simulink model "AWD_EV_MODEL_rev2"  (Simulink 8.7)
settings: Solver=ode3  SolverMode=SingleTasking  StartTime=0.0  StopTime=20  FixedStep=0.001  RelTol=1e-3
undefined symbols (not defined in the file): Bx, Bx_2, By, By_2, Cx, Cx_2, Cy, Cy_2, Dx, Dx_2, Dy, Dy_2, Ex, Ex_2, Ey, Ey_2, g, GRR, GRR_E, hg, Ixx, Iyy, Jw, Jz, Lf, Lr, Lw, m, r0, Rw, rx1, rx1_2, rx2, rx2_2, ry1, ry1_2, ry2, ry2_2, SA_A, SA_SAT_n, SA_SAT_p, SA_Slope, sigbuilder_block, Split_u_Time_On, SR_Eq_Accel_Brake_Threshold, Steering_Input_Select, T_Avail, Throttle_Final_Val, Throttle_Init_Val, Throttle_Step_Time, Vx0, Vy0, wRL0, z
libraries: simulink x10
(part 1 of 2)
settings Model: Creator=ETLAB  LastModifiedBy=MR Spyder
settings DataIOCC: SignalLoggingSaveFormat=ModelDataLogs
settings OptimizationCC: ExpressionDepthLimit=2147483647
settings DebuggingCC: SolverPrmCheckMsg=warning  InheritedTsInSrcMsg=none  FcnCallInpInsideContextMsg=EnableAllAsWarning  StateNameClashWarn=warning
settings GRTTargetCC: CombineOutputUpdateFcns=off  GRTInterface=on

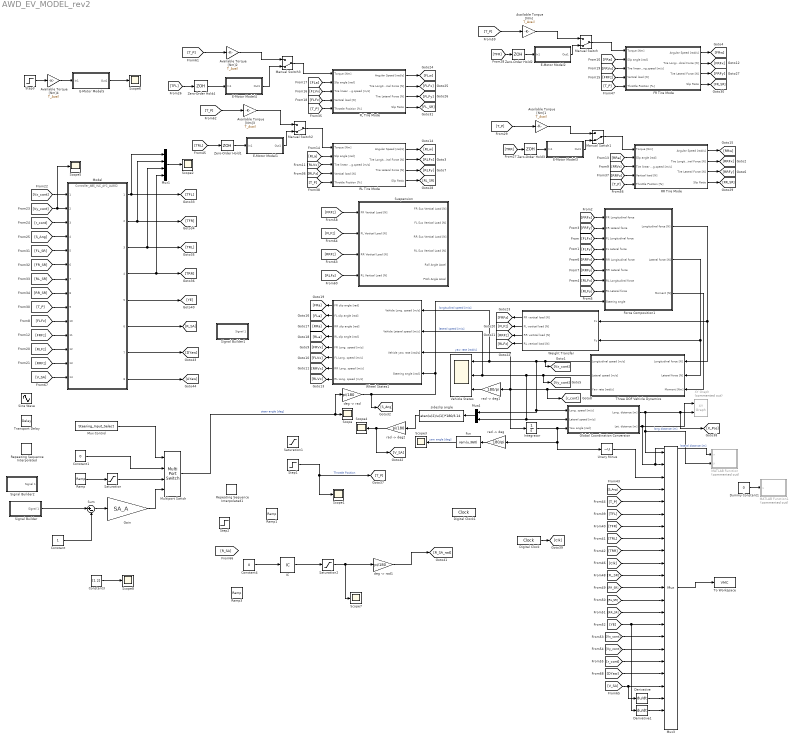
== system AWD_EV_MODEL_rev2 ==
  Available Torque [Nm]{,1..4} (5 alike) : Gain  Gain=T_Avail
  Constant : Constant
  Constant1 : Constant  Value=0
  Constant3 : Constant  Value=[1 2]
  Constant4 : Constant  Value=0
  Derivative : Derivative
  Derivative1 : Derivative
  Digital Clock : DigitalClock  SampleTime=0.001
  Digital Clock1 : DigitalClock  SampleTime=0.001
  Dummy Constant1 : Constant  Value=0
  E-Motor Model1 : Subsystem
  E-Motor Model2 : Subsystem
  E-Motor Model3 : Subsystem
  E-Motor Model4 : Subsystem
  E-Motor Model5 : Subsystem
  FL Tire Mode : Subsystem
      mask Display:
      | image(imread('Tire.bmp'),'center')
      | port_label('input', 1, 'Torque [Nm]')
      | port_label('input', 2, 'Slip angle [rad]')
      | port_label('input', 3, 'Long. speed [m/s]')
      | port_label('input', 4, 'Vertical load [N]')
      | port_label('input', 5, 'Throttle Position [%]')
      | port_label('output', 1, 'Angular speed [rad/s]')
      | port_label('output', 2, 'Long. force [N]')
      | port_label('output', 3, 'Lateral force [N]')
      | port_label('output', 4, 'Slip Ratio')
  FR Tire Mode : Subsystem
      mask Display:
      | image(imread('Tire.bmp'),'center')
      | port_label('input', 1, 'Torque [Nm]')
      | port_label('input', 2, 'Slip angle [rad]')
      | port_label('input', 3, 'Long. speed [m/s]')
      | port_label('input', 4, 'Vertical load [N]')
      | port_label('input', 5, 'Throttle Position [%]')
      | port_label('output', 1, 'Angular speed [rad/s]')
      | port_label('output', 2, 'Long. force [N]')
      | port_label('output', 3, 'Lateral force [N]')
      | port_label('output', 4, 'Slip Ratio')
  Fcn : Fcn  Expr=rem(u,360)
  Force Composition1 : Subsystem
  Gain : Gain  Gain=SA_A
  Global Coordination Conversion : Subsystem
  IC : InitialCondition  Value=0
  Integrator : Integrator
  MATLAB Function : MATLAB Function  Commented=on  TreatAsAtomicUnit=on
  MATLAB Function1 : MATLAB Function  Commented=on  TreatAsAtomicUnit=on
  Manual Switch{,1..3} (4 alike) : ManualSwitch  CurrentSetting=0
  Model : ModelReference  ModelNameDialog=Controller_ABS_VLC_AYC_ALGO2.mdl  SimulationMode=Normal  ModelReferenceVersion=1.794
  Multiport Switch : MultiPortSwitch
  Mux Control : Constant  Value=Steering_Input_Select
  Mux1 : Mux
  Mux3 : Mux  Inputs=23
  Mux4 : Mux  Inputs=2
  RL Tire Mode : Subsystem
      mask Display:
      | image(imread('Tire.bmp'),'center')
      | port_label('input', 1, 'Torque [Nm]')
      | port_label('input', 2, 'Slip angle [rad]')
      | port_label('input', 3, 'Long. speed [m/s]')
      | port_label('input', 4, 'Vertical load [N]')
      | port_label('input', 5, 'Throttle Position [%]')
      | port_label('output', 1, 'Angular speed [rad/s]')
      | port_label('output', 2, 'Long. force [N]')
      | port_label('output', 3, 'Lateral force [N]')
      | port_label('output', 4, 'Slip Ratio')
  RR Tire Mode : Subsystem
      mask Display:
      | image(imread('Tire.bmp'),'center')
      | port_label('input', 1, 'Torque [Nm]')
      | port_label('input', 2, 'Slip angle [rad]')
      | port_label('input', 3, 'Long. speed [m/s]')
      | port_label('input', 4, 'Vertical load [N]')
      | port_label('input', 5, 'Throttle Position [%]')
      | port_label('output', 1, 'Angular speed [rad/s]')
      | port_label('output', 2, 'Long. force [N]')
      | port_label('output', 3, 'Lateral force [N]')
  Ramp : simulink/Sources/Ramp  slope=SA_Slope  start=SA_Start_Time  X0=0
  Ramp1 : simulink/Sources/Ramp  slope=10  start=.02  X0=-1
  Ramp3 : simulink/Sources/Ramp  slope=0.5  start=11  X0=0
  Repeating Sequence Interpolated : simulink/Sources/Repeating Sequence Interpolated  OutValues=[0 0 7 0 0 -7 0 0].'  TimeValues=[0 2 4 6 8 10 26 28].'  LookUpMeth=Interpolation-Use End Values  tsamp=0.001  OutMin=[]  OutMax=[]  OutDataTypeStr=double  OutputDataTypeScalingMode=double  OutDataType=fixdt(0,8)  OutScaling=2^-10
  Repeating Sequence Interpolated1 : simulink/Sources/Repeating Sequence Interpolated  OutValues=[-0.99 -0.99 -0.3 -0.3 -0.5 -0.5].'  TimeValues=[0 0.5 1.1 2 2.1 10].'  LookUpMeth=Interpolation-Use End Values  tsamp=0.001  OutMin=[]  OutMax=[]  OutDataTypeStr=double  OutputDataTypeScalingMode=double  OutDataType=fixdt(0,8)  OutScaling=2^-10
  Saturation : Saturate  UpperLimit=SA_SAT_p  LowerLimit=SA_SAT_n
  Saturation1 : Saturate  UpperLimit=1  LowerLimit=-1
  Saturation2 : Saturate  UpperLimit=5  LowerLimit=-5
  Scope{,1..8} (9 alike) : Scope
  Signal Builder : Subsystem  Tag=STV Subsys  LoadFcn=sigbuilder_block('load');  StartFcn=sigbuilder_block('start');  StopFcn=sigbuilder_block('stop');  ClipboardFcn=sigbuilder_block('clipboard');  mask(Sigbuilder block){}
      mask help: Simulink:masks:SigbuilderBlock_MD
      mask init:
      | if ~strcmp(get_param(bdroot(gcbh),'SimulationStatus'),'stopped') tuvar = sigbuilder_block('maskInit'); end
      settings: CopyFcn=sigbuilder_block('copy');  DeleteFcn=sigbuilder_block('delete');  ModelCloseFcn=sigbuilder_block('modelClose');  PreSaveFcn=sigbuilder_block('preSave');  PauseFcn=sigbuilder_block('pause');  ContinueFcn=sigbuilder_block('continue');  NameChangeFcn=sigbuilder_block('namechange');  OpenFcn=sigbuilder_block('open',[3 41.25 1428 682.5 ]);  CloseFcn=sigbuilder_block('close');
      mask Display: plot(0, 0, 100, 100,[2, 2, 32, 32, 2], [68, 8, 8, 68, 68],[32, 2], [38, 38], [32, 19, 2],[53, 60, 44], [32, 17, 17, 2],[16, 16, 31, 31]);txt = getActiveGroup(gcbh);text(2, 100, txt,'verticalAlignment', 'top');
  Signal Builder1 : Subsystem  Tag=STV Subsys  LoadFcn=sigbuilder_block('load');  StartFcn=sigbuilder_block('start');  StopFcn=sigbuilder_block('stop');  ClipboardFcn=sigbuilder_block('clipboard');  mask(Sigbuilder block){}
      mask help: Simulink:masks:SigbuilderBlock_MD
      mask init:
      | if ~strcmp(get_param(bdroot(gcbh),'SimulationStatus'),'stopped') tuvar = sigbuilder_block('maskInit'); end
      settings: CopyFcn=sigbuilder_block('copy');  DeleteFcn=sigbuilder_block('delete');  ModelCloseFcn=sigbuilder_block('modelClose');  PreSaveFcn=sigbuilder_block('preSave');  PauseFcn=sigbuilder_block('pause');  ContinueFcn=sigbuilder_block('continue');  NameChangeFcn=sigbuilder_block('namechange');  OpenFcn=sigbuilder_block('open',[6 36 1428 711 ]);  CloseFcn=sigbuilder_block('close');
      mask Display: plot(0, 0, 100, 100,[2, 2, 32, 32, 2], [68, 8, 8, 68, 68],[32, 2], [38, 38], [32, 19, 2],[53, 60, 44], [32, 17, 17, 2],[16, 16, 31, 31]);txt = getActiveGroup(gcbh);text(2, 100, txt,'verticalAlignment', 'top');
  Signal Builder2 : Subsystem  Tag=STV Subsys  LoadFcn=sigbuilder_block('load');  StartFcn=sigbuilder_block('start');  StopFcn=sigbuilder_block('stop');  ClipboardFcn=sigbuilder_block('clipboard');  mask(Sigbuilder block){}
      mask help: Simulink:masks:SigbuilderBlock_MD
      mask init:
      | if ~strcmp(get_param(bdroot(gcbh),'SimulationStatus'),'stopped') tuvar = sigbuilder_block('maskInit'); end
      settings: CopyFcn=sigbuilder_block('copy');  DeleteFcn=sigbuilder_block('delete');  ModelCloseFcn=sigbuilder_block('modelClose');  PreSaveFcn=sigbuilder_block('preSave');  PauseFcn=sigbuilder_block('pause');  ContinueFcn=sigbuilder_block('continue');  NameChangeFcn=sigbuilder_block('namechange');  OpenFcn=sigbuilder_block('open',[6 30 1428 682.5 ]);  CloseFcn=sigbuilder_block('close');
      mask Display: plot(0, 0, 100, 100,[2, 2, 32, 32, 2], [68, 8, 8, 68, 68],[32, 2], [38, 38], [32, 19, 2],[53, 60, 44], [32, 17, 17, 2],[16, 16, 31, 31]);txt = getActiveGroup(gcbh);text(2, 100, txt,'verticalAlignment', 'top');
  Sine Wave : Sin  Amplitude=4  Frequency=.1  SampleTime=0
  Step1 : Step  Time=Throttle_Step_Time  Before=Throttle_Init_Val  After=Throttle_Final_Val  SampleTime=0
  Step2 : Step  Time=Throttle_Step_Time  Before=Throttle_Init_Val  After=Throttle_Final_Val  SampleTime=0
  Step3 : Step  SampleTime=0
  Sum : Sum  Inputs=|+-
  Suspension : Subsystem
  Three DOF Vehicle Dynamics : Subsystem
      mask Display:
      | image(imread('Vehicle.bmp'),'center')
      | port_label('input', 1, 'Longitudinal force [N]')
      | port_label('input', 2, 'Lateral force [N]')
      | port_label('input', 3, 'Moment [Nm]')
      | port_label('output', 1, 'Longitudinal speed [m/s]')
      | port_label('output', 2, 'Lateral speed [m/s]')
      | port_label('output', 3, 'Yaw rate [rad/s]')
  To Workspace : ToWorkspace  VariableName=VMC  SampleTime=-1
  Transport Delay : TransportDelay  DelayTime=.5
  Unary Minus : UnaryMinus
  Vehicle States : Scope  NumInputPorts=3
  Weight Transfer : Subsystem
  Wheel States1 : Subsystem
  XY Graph : simulink/Sinks/XY Graph  Commented=on  xmin=-500  xmax=500  ymin=-500  ymax=500  st=-1
  Zero-Order Hold{1..4} (4 alike) : ZeroOrderHold  SampleTime=.001
  "deg -> rad" : Gain  Gain=pi/180
  "deg -> rad1" : Gain  Gain=pi/180
  "rad -> deg" : Gain  Gain=180/pi
  "rad -> deg1" : Gain  Gain=180/pi
  "rad -> deg2" : Gain  Gain=pi/180
  sideslip angle : Fcn  Expr=atan(u(2)/u(1))*180/3.14
  wires:
  Wheel States1/5(FR Long. speed [m/s]) -> [FRVx]
  Wheel States1/6(FL Long. speed [m/s]) -> [FLVx]
  Wheel States1/7(RR Long. speed [m/s]) -> [RRVx]
  Wheel States1/8(RL Long. speed [m/s]) -> [RLVx]
  Three DOF Vehicle Dynamics/3(Yaw rate [rad/s]) -> Wheel States1/3(Vehicle yaw rate [rad/s]), "rad -> deg1"/1, Integrator/1, [r_cont]  "yaw rate [rad/s]"
  Three DOF Vehicle Dynamics/2(Lateral speed [m/s]) -> Wheel States1/2(Vehicle Lateral speed [m/s]), Vehicle States/2, Global Coordination Conversion/2(Lateral speed [m/s]), Mux4/2, [Vy_cont]  "lateral speed [m/s]"
  Three DOF Vehicle Dynamics/1(Longitudinal speed [m/s]) -> Wheel States1/1(Vehicle Long. speed [m/s]), Vehicle States/1, Global Coordination Conversion/1(Long. speed [m/s]), Mux4/1, [Vx_cont]  "longitudinal speed [m/s]"
  Wheel States1/1("FR slip angle [rad] ") -> [FRa]
  Wheel States1/2("FL slip angle [rad] ") -> [FLa]
  Wheel States1/3("RR slip angle [rad] ") -> [RRa]
  Wheel States1/4("RL slip angle [rad] ") -> [RLa]
  Force Composition1/1(Longitudinal force [N]) -> Weight Transfer/1(Fx), Three DOF Vehicle Dynamics/1(Longitudinal force [N])
  [FRFx] -> Force Composition1/1(FR Longitudinal force)
  [FRFy] -> Force Composition1/2(FR Lateral force)
  [FLFx] -> Force Composition1/3(FL Longitudinal force)
  [FLFy] -> Force Composition1/4(FL Lateral force)
  [RRFx] -> Force Composition1/5(RR Longitudinal force)
  [RRFy] -> Force Composition1/6(RR Lateral force)
  [RLFx] -> Force Composition1/7(RL Longitudinal force)
  [RLFy] -> Force Composition1/8(RL Lateral force)
  "rad -> deg"/1 -> Fcn/1
  Fcn/1 -> Scope3/1  "yaw angle [deg]"
  Global Coordination Conversion/1(Long. distance [m]) -> MATLAB Function/2(y), Mux3/1, XY Graph/2, [X_Pos]  "long distance [m]"
  Global Coordination Conversion/2(Lat. distance [m]) -> XY Graph/1, MATLAB Function/1(x), Mux3/2  "lateral distance [m]"
  Weight Transfer/1(FR vertical load [N]) -> [FRFz]
  Weight Transfer/2(FL vertical load [N]) -> [FLFz]
  Weight Transfer/3(RR vertical load [N]) -> [RRFz]
  Weight Transfer/4(RL vertical load [N]) -> [RLFz]
  Force Composition1/2(Lateral force [N]) -> Weight Transfer/2(Fy), Three DOF Vehicle Dynamics/2(Lateral force [N])
  Integrator/1 -> Global Coordination Conversion/3(Yaw angle [rad]), "rad -> deg"/1, Unary Minus/1
  Force Composition1/3(Moment [N]) -> Three DOF Vehicle Dynamics/3(Moment [Nm])
  "rad -> deg1"/1 -> Vehicle States/3
  Mux4/1 -> sideslip angle/1
  sideslip angle/1 -> "rad -> deg2"/1
  FL Tire Mode/2(Tire Longitudinal Force [N]) -> [FLFx]
  FL Tire Mode/1(Angular Speed [rad/s]) -> [FLw]
  [FLVx] -> FL Tire Mode/3(Tire linear Long.speed [m/s])
  [FLa] -> FL Tire Mode/2(Slip angle [rad])
  [FLFz] -> FL Tire Mode/4(Vertical load [N])
  FL Tire Mode/3(Tire Lateral Force [N]) -> [FLFy]
  FL Tire Mode/4(Slip Ratio) -> [FL_SR]
  Mux3/1 -> To Workspace/1
  [FRa] -> FR Tire Mode/2(Slip angle [rad])
  [FRVx] -> FR Tire Mode/3(Tire linear Long.speed [m/s])
  [FRFz] -> FR Tire Mode/4(Vertical load [N])
  FR Tire Mode/1(Angular Speed [rad/s]) -> [FRw]
  FR Tire Mode/2(Tire Longitudinal Force [N]) -> [FRFx]
  FR Tire Mode/3(Tire Lateral Force [N]) -> [FRFy]
  FR Tire Mode/4(Slip Ratio) -> [FR_SR]
  [RLa] -> RL Tire Mode/2(Slip angle [rad])
  [RLVx] -> RL Tire Mode/3(Tire linear Long.speed [m/s])
  [RLFz] -> RL Tire Mode/4(Vertical load [N])
  RL Tire Mode/1(Angular Speed [rad/s]) -> [RLw]
  RL Tire Mode/2(Tire Longitudinal Force [N]) -> [RLFx]
  RL Tire Mode/3(Tire Lateral Force [N]) -> [RLFy]
  RL Tire Mode/4(Slip Ratio) -> [RL_SR]
  [RRa] -> RR Tire Mode/2(Slip angle [rad])
  [RRVx] -> RR Tire Mode/3(Tire linear Long.speed [m/s])
  [RRFz] -> RR Tire Mode/4(Vertical load [N])
  RR Tire Mode/1(Angular Speed [rad/s]) -> [RRw]
  RR Tire Mode/2(Tire Longitudinal Force [N]) -> [RRFx]
  RR Tire Mode/3(Tire Lateral Force [N]) -> [RRFy]
  RR Tire Mode/4(Slip Ratio) -> [RR_SR]
  "deg -> rad"/1 -> [S_Ang], Force Composition1/9(Steering angle), Wheel States1/4(Steering angle [rad])
  Unary Minus/1 -> Mux3/3
  Step1/1 -> Scope1/1, [T_P]  "Throttle Position"
  [Vx_cont] -> Model/1
  [Vy_cont] -> Model/2, Scope5/1
  [r_cont] -> Model/3
  [S_Ang] -> Model/4
  [FL_SR] -> Model/5
  [FR_SR] -> Model/6
  [RL_SR] -> Model/7
  [RR_SR] -> Model/8
  [T_P] -> Model/9
  [T_P] -> FL Tire Mode/5(Throttle Position [%])
  [T_P] -> RL Tire Mode/5(Throttle Position [%])
  [S_Ang] -> Mux3/4
  [TFL] -> Mux3/6
  [TFR] -> Mux3/7
  [TRL] -> Mux3/8
  [TRR] -> Mux3/9
  [T_P] -> Mux3/5
  [Clk] -> Mux3/10
  Digital Clock/1 -> [Clk]
  Model/1 -> Mux1/1, [TFL]
  Model/2 -> Mux1/2, [TFR]
  Model/3 -> Mux1/3, [TRL]
  Model/4 -> Mux1/4, [TRR]
  Manual Switch3/1 -> FL Tire Mode/1(Torque [Nm])
  Manual Switch1/1 -> RR Tire Mode/1(Torque [Nm])
  Manual Switch/1 -> FR Tire Mode/1(Torque [Nm])
  [FL_SR] -> Mux3/11
  [FR_SR] -> Mux3/12
  [RL_SR] -> Mux3/13
  [RR_SR] -> Mux3/14
  Model/5 -> [YE]
  [YE] -> Mux3/15, Derivative1/1
  [Vx_cont] -> Mux3/16
  [Vy_cont] -> Mux3/17
  [r_cont] -> Mux3/18
  Dummy Constant1/1 -> MATLAB Function1/1(u)
  [FLFz] -> Model/10
  [FRFz] -> Model/11
  [RLFz] -> Model/12
  [RRFz] -> Model/13
  Mux Control/1 -> Multiport Switch/1
  Ramp/1 -> Saturation/1
  Constant1/1 -> Multiport Switch/2
  [T_P] -> FR Tire Mode/5(Throttle Position [%])
  [T_P] -> RR Tire Mode/5(Throttle Position [%])
  [DYaw] -> Mux3/19
  Mux1/1 -> Scope2/1
  Manual Switch2/1 -> RL Tire Mode/1(Torque [Nm])
  Zero-Order Hold4/1 -> E-Motor Model4/1(In1)
  [TFL] -> Zero-Order Hold4/1
  E-Motor Model4/1(Out1) -> Manual Switch3/2
  Available Torque [Nm]2/1 -> Manual Switch3/1
  [T_P] -> Available Torque [Nm]2/1
  Zero-Order Hold1/1 -> E-Motor Model1/1(In1)
  [TRL] -> Zero-Order Hold1/1
  E-Motor Model1/1(Out1) -> Manual Switch2/2
  Available Torque [Nm]3/1 -> Manual Switch2/1
  [T_P] -> Available Torque [Nm]3/1
  Zero-Order Hold2/1 -> E-Motor Model2/1(In1)
  [TFR] -> Zero-Order Hold2/1
  E-Motor Model2/1(Out1) -> Manual Switch/2
  Available Torque [Nm]/1 -> Manual Switch/1
  [T_P] -> Available Torque [Nm]/1
  Zero-Order Hold3/1 -> E-Motor Model3/1(In1)
  [TRR] -> Zero-Order Hold3/1
  E-Motor Model3/1(Out1) -> Manual Switch1/2
  Available Torque [Nm]1/1 -> Manual Switch1/1
  [T_P] -> Available Torque [Nm]1/1
  [FLFz] -> Suspension/2(FL Vertical Load [N])
  [FRFz] -> Suspension/1(FR Vertical Load [N])
  [RLFz] -> Suspension/4(RL Vertical Load [N])
  [RRFz] -> Suspension/3(RR Vertical Load [N])
  Step3/1 -> Available Torque [Nm]4/1
  E-Motor Model5/1(Out1) -> Scope6/1
  Available Torque [Nm]4/1 -> E-Motor Model5/1(In1)
  "deg -> rad1"/1 -> [R_SA_rad]
  Saturation2/1 -> Scope7/1, "deg -> rad1"/1
  Multiport Switch/1 -> "deg -> rad"/1, Scope/1  "steer angle [deg]"
  Gain/1 -> Multiport Switch/4
  Sum/1 -> Gain/1
  Constant/1 -> Sum/2
  [V_SA] -> Derivative/1, Mux3/20
  Model/6 -> [R_SA]
  IC/1 -> Saturation2/1
  Constant4/1 -> IC/1
  [V_SA] -> Model/14
  Constant3/1 -> Scope8/1
  "rad -> deg2"/1 -> [V_SA], Scope4/1
  Signal Builder/1(Signal 1) -> Sum/1
  Saturation/1 -> Multiport Switch/3
  Model/7 -> [DYaw]
  Model/8 -> [AYaw]
  Derivative/1 -> Mux3/21
  Derivative1/1 -> Mux3/22

== system AWD_EV_MODEL_rev2/E-Motor Model1 ==
  In1 : Inport
  Digital Clock : DigitalClock  SampleTime=0.001
  Switch1 : Switch  Threshold=.02
  Transfer Fcn : TransferFcn  Denominator=[2*z*z 2*z 1]
  Out1 : Outport
  wires:
  In1/1 -> Transfer Fcn/1, Switch1/3
  Digital Clock/1 -> Switch1/2
  Transfer Fcn/1 -> Switch1/1
  Switch1/1 -> Out1/1

== system AWD_EV_MODEL_rev2/E-Motor Model2 ==
  In1 : Inport
  Digital Clock : DigitalClock  SampleTime=0.001
  Switch1 : Switch  Threshold=.02
  Transfer Fcn : TransferFcn  Denominator=[2*z*z 2*z 1]
  Out1 : Outport
  wires:
  In1/1 -> Transfer Fcn/1, Switch1/3
  Digital Clock/1 -> Switch1/2
  Transfer Fcn/1 -> Switch1/1
  Switch1/1 -> Out1/1

== system AWD_EV_MODEL_rev2/E-Motor Model3 ==
  In1 : Inport
  Digital Clock : DigitalClock  SampleTime=0.001
  Switch1 : Switch  Threshold=.02
  Transfer Fcn : TransferFcn  Denominator=[2*z*z 2*z 1]
  Out1 : Outport
  wires:
  In1/1 -> Transfer Fcn/1, Switch1/3
  Digital Clock/1 -> Switch1/2
  Transfer Fcn/1 -> Switch1/1
  Switch1/1 -> Out1/1

== system AWD_EV_MODEL_rev2/E-Motor Model4 ==
  In1 : Inport
  Digital Clock : DigitalClock  SampleTime=0.001
  Switch1 : Switch  Threshold=.02
  Transfer Fcn : TransferFcn  Denominator=[2*z*z 2*z 1]
  Out1 : Outport
  wires:
  In1/1 -> Transfer Fcn/1, Switch1/3
  Digital Clock/1 -> Switch1/2
  Transfer Fcn/1 -> Switch1/1
  Switch1/1 -> Out1/1

== system AWD_EV_MODEL_rev2/E-Motor Model5 ==
  In1 : Inport
  Digital Clock : DigitalClock  SampleTime=0.001
  Switch1 : Switch  Threshold=.02
  Transfer Fcn : TransferFcn  Denominator=[2*z*z 2*z 1]
  Out1 : Outport
  wires:
  In1/1 -> Transfer Fcn/1, Switch1/3
  Digital Clock/1 -> Switch1/2
  Transfer Fcn/1 -> Switch1/1
  Switch1/1 -> Out1/1

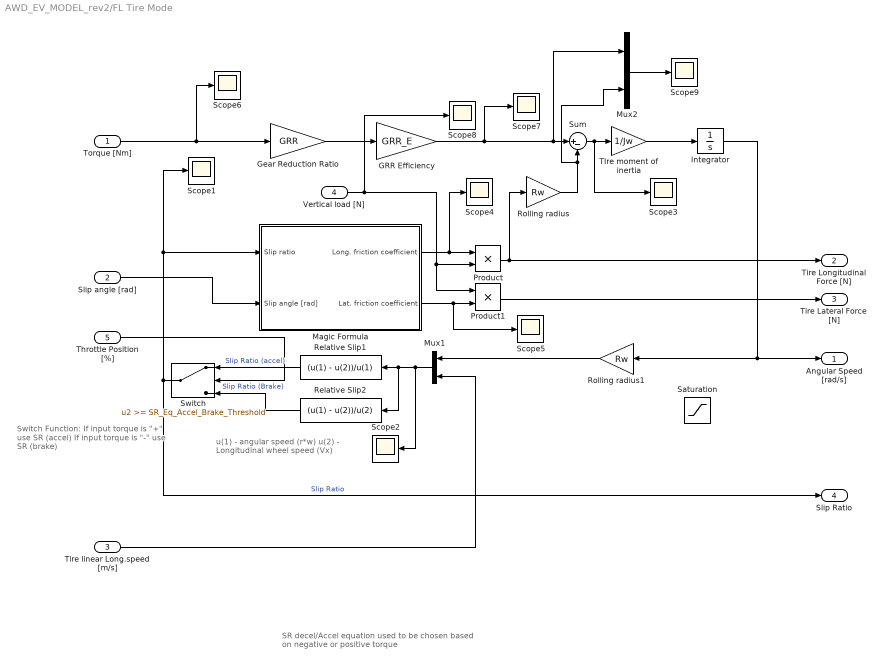
== system AWD_EV_MODEL_rev2/FL Tire Mode ==
  note: SR decel/Accel equation used to be chosen
      | based on negative or positive torque
  note: u(1) - angular speed (r*w)
      | u(2) - Longitudinal wheel speed (Vx)
  note: Switch Function:
      | If input torque is "+" use SR (accel)
      | If input torque is "-" use SR (brake)
  Torque [Nm] : Inport
  Slip angle [rad] : Inport  Port=2
  Tire linear Long.speed [m/s] : Inport  Port=3
  Vertical load [N] : Inport  Port=4
  Throttle Position [%] : Inport  Port=5
  GRR Efficiency : Gain  Gain=GRR_E  SaturateOnIntegerOverflow=on  OutDataTypeStr=Inherit: Same as input  ParamDataTypeStr=Inherit: Same as input
  Gear Reduction Ratio : Gain  Gain=GRR  SaturateOnIntegerOverflow=on  OutDataTypeStr=Inherit: Same as input  ParamDataTypeStr=Inherit: Same as input
  Integrator : Integrator  InitialCondition=wRL0
  Magic Formula : Subsystem  mask(Magic Formula (Combined Slip)){}
      mask Display:
      | image(imread('Magic formula.jpg'),'center')
      | port_label('input', 1, 'slip ratio')
      | port_label('input', 2, 'slip angle')
      | port_label('output', 1, 'Mux')
      | port_label('output', 2, 'Muy')
  Mux1 : Mux  Inputs=2
  Mux2 : Mux  Inputs=2
  Product : Product  RndMeth=Zero
  Product1 : Product  RndMeth=Zero
  Relative Slip1 : Fcn  Expr=(u(1) - u(2))/u(1)
  Relative Slip2 : Fcn  Expr=(u(1) - u(2))/u(2)
  Rolling radius : Gain  Gain=Rw  SaturateOnIntegerOverflow=on  OutDataTypeStr=Inherit: Same as input  ParamDataTypeStr=Inherit: Same as input
  Rolling radius1 : Gain  Gain=Rw  SaturateOnIntegerOverflow=on  OutDataTypeStr=Inherit: Same as input  ParamDataTypeStr=Inherit: Same as input
  Saturation : Saturate  UpperLimit=1000  LowerLimit=0.00001
  Scope{1..9} (9 alike) : Scope
  Sum : Sum  Inputs=|+-
  Switch : Switch  Threshold=SR_Eq_Accel_Brake_Threshold
  TIre moment of inertia : Gain  Gain=1/Jw  SaturateOnIntegerOverflow=on  OutDataTypeStr=Inherit: Same as input  ParamDataTypeStr=Inherit: Same as input
  Angular Speed [rad/s] : Outport
  Tire Longitudinal Force [N] : Outport  Port=2
  Tire Lateral Force [N] : Outport  Port=3
  Slip Ratio : Outport  Port=4
  wires:
  Slip angle [rad]/1 -> Magic Formula/2(Slip angle [rad])
  Tire linear Long.speed [m/s]/1 -> Mux1/2
  Torque [Nm]/1 -> Scope6/1, Gear Reduction Ratio/1
  Sum/1 -> TIre moment of inertia/1, Scope3/1
  TIre moment of inertia/1 -> Integrator/1
  Rolling radius/1 -> Mux2/2, Sum/2
  Mux1/1 -> Scope2/1, Relative Slip1/1, Relative Slip2/1
  Rolling radius1/1 -> Mux1/1
  Magic Formula/1(Long. friction coefficient) -> Product/1, Scope4/1
  Magic Formula/2(Lat. friction coefficient) -> Product1/2, Scope5/1
  Product/1 -> Rolling radius/1, Tire Longitudinal Force [N]/1
  Vertical load [N]/1 -> Product/2, Product1/1, Scope8/1
  Product1/1 -> Tire Lateral Force [N]/1
  Gear Reduction Ratio/1 -> GRR Efficiency/1
  GRR Efficiency/1 -> Scope7/1, Mux2/1, Sum/1
  Relative Slip1/1 -> Switch/1  "Slip Ratio (accel)"
  Relative Slip2/1 -> Switch/3  "Slip Ratio (Brake)"
  Switch/1 -> Scope1/1, Magic Formula/1(Slip ratio), Slip Ratio/1  "Slip Ratio"
  Mux2/1 -> Scope9/1
  Throttle Position [%]/1 -> Switch/2
  Integrator/1 -> Rolling radius1/1, Angular Speed [rad/s]/1

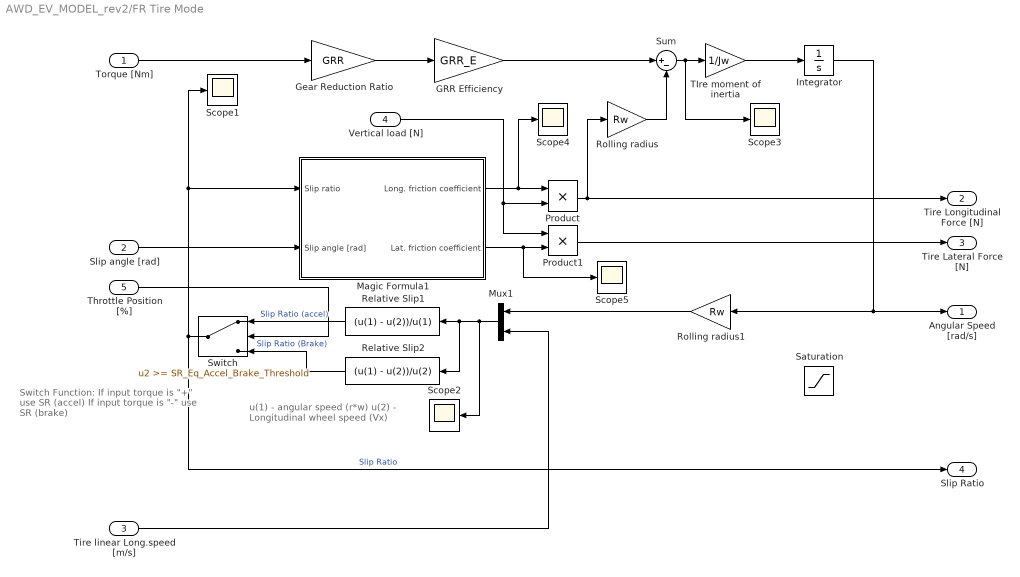
== system AWD_EV_MODEL_rev2/FR Tire Mode ==
  note: u(1) - angular speed (r*w)
      | u(2) - Longitudinal wheel speed (Vx)
  note: Switch Function:
      | If input torque is "+" use SR (accel)
      | If input torque is "-" use SR (brake)
  Torque [Nm] : Inport
  Slip angle [rad] : Inport  Port=2
  Tire linear Long.speed [m/s] : Inport  Port=3
  Vertical load [N] : Inport  Port=4
  Throttle Position [%] : Inport  Port=5
  GRR Efficiency : Gain  Gain=GRR_E  SaturateOnIntegerOverflow=on  OutDataTypeStr=Inherit: Same as input  ParamDataTypeStr=Inherit: Same as input
  Gear Reduction Ratio : Gain  Gain=GRR  SaturateOnIntegerOverflow=on  OutDataTypeStr=Inherit: Same as input  ParamDataTypeStr=Inherit: Same as input
  Integrator : Integrator  InitialCondition=wRL0
  Magic Formula1 : Subsystem  mask(Magic Formula (Combined Slip)){}
      mask Display:
      | image(imread('Magic formula.jpg'),'center')
      | port_label('input', 1, 'slip ratio')
      | port_label('input', 2, 'slip angle')
      | port_label('output', 1, 'Mux')
      | port_label('output', 2, 'Muy')
  Mux1 : Mux  Inputs=2
  Product : Product  RndMeth=Zero
  Product1 : Product  RndMeth=Zero
  Relative Slip1 : Fcn  Expr=(u(1) - u(2))/u(1)
  Relative Slip2 : Fcn  Expr=(u(1) - u(2))/u(2)
  Rolling radius : Gain  Gain=Rw  SaturateOnIntegerOverflow=on  OutDataTypeStr=Inherit: Same as input  ParamDataTypeStr=Inherit: Same as input
  Rolling radius1 : Gain  Gain=Rw  SaturateOnIntegerOverflow=on  OutDataTypeStr=Inherit: Same as input  ParamDataTypeStr=Inherit: Same as input
  Saturation : Saturate  UpperLimit=1000  LowerLimit=0.00001
  Scope{1..5} (5 alike) : Scope
  Sum : Sum  Inputs=|+-
  Switch : Switch  Threshold=SR_Eq_Accel_Brake_Threshold
  TIre moment of inertia : Gain  Gain=1/Jw  SaturateOnIntegerOverflow=on  OutDataTypeStr=Inherit: Same as input  ParamDataTypeStr=Inherit: Same as input
  Angular Speed [rad/s] : Outport
  Tire Longitudinal Force [N] : Outport  Port=2
  Tire Lateral Force [N] : Outport  Port=3
  Slip Ratio : Outport  Port=4
  wires:
  Slip angle [rad]/1 -> Magic Formula1/2(Slip angle [rad])
  Tire linear Long.speed [m/s]/1 -> Mux1/2
  Torque [Nm]/1 -> Gear Reduction Ratio/1
  Sum/1 -> TIre moment of inertia/1, Scope3/1
  TIre moment of inertia/1 -> Integrator/1
  Rolling radius/1 -> Sum/2
  Mux1/1 -> Scope2/1, Relative Slip1/1, Relative Slip2/1
  Rolling radius1/1 -> Mux1/1
  Magic Formula1/1(Long. friction coefficient) -> Product/1, Scope4/1
  Magic Formula1/2(Lat. friction coefficient) -> Product1/2, Scope5/1
  Product/1 -> Rolling radius/1, Tire Longitudinal Force [N]/1
  Vertical load [N]/1 -> Product/2, Product1/1
  Product1/1 -> Tire Lateral Force [N]/1
  Gear Reduction Ratio/1 -> GRR Efficiency/1
  GRR Efficiency/1 -> Sum/1
  Relative Slip1/1 -> Switch/1  "Slip Ratio (accel)"
  Relative Slip2/1 -> Switch/3  "Slip Ratio (Brake)"
  Switch/1 -> Magic Formula1/1(Slip ratio), Scope1/1, Slip Ratio/1  "Slip Ratio"
  Throttle Position [%]/1 -> Switch/2
  Integrator/1 -> Rolling radius1/1, Angular Speed [rad/s]/1

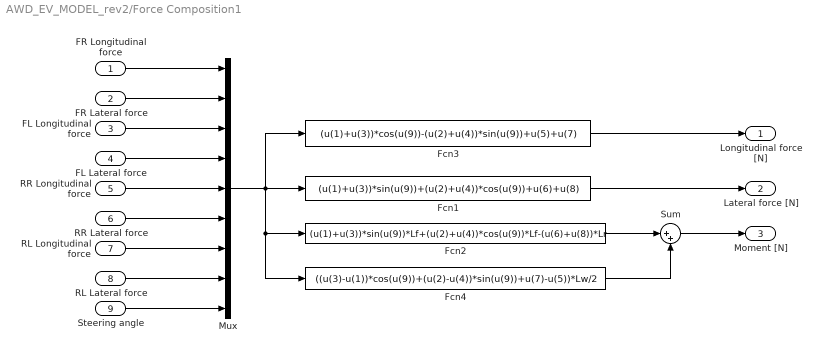
== system AWD_EV_MODEL_rev2/Force Composition1 ==
  FR Longitudinal force : Inport
  FR Lateral force : Inport  Port=2
  FL Longitudinal force : Inport  Port=3
  FL Lateral force : Inport  Port=4
  RR Longitudinal force : Inport  Port=5
  RR Lateral force : Inport  Port=6
  RL Longitudinal force : Inport  Port=7
  RL Lateral force : Inport  Port=8
  Steering angle : Inport  Port=9
  Fcn1 : Fcn  Expr=(u(1)+u(3))*sin(u(9))+(u(2)+u(4))*cos(u(9))+u(6)+u(8)
  Fcn2 : Fcn  Expr=(u(1)+u(3))*sin(u(9))*Lf+(u(2)+u(4))*cos(u(9))*Lf-(u(6)+u(8))*Lr
  Fcn3 : Fcn  Expr=(u(1)+u(3))*cos(u(9))-(u(2)+u(4))*sin(u(9))+u(5)+u(7)
  Fcn4 : Fcn  Expr=((u(3)-u(1))*cos(u(9))+(u(2)-u(4))*sin(u(9))+u(7)-u(5))*Lw/2
  Mux : Mux  Inputs=9
  Sum : Sum  Inputs=|++
  Longitudinal force [N] : Outport
  Lateral force [N] : Outport  Port=2
  Moment [N] : Outport  Port=3
  wires:
  Mux/1 -> Fcn3/1, Fcn1/1, Fcn2/1, Fcn4/1
  Fcn3/1 -> Longitudinal force [N]/1
  Fcn1/1 -> Lateral force [N]/1
  Sum/1 -> Moment [N]/1
  Fcn2/1 -> Sum/1
  Fcn4/1 -> Sum/2
  FR Longitudinal force/1 -> Mux/1
  FR Lateral force/1 -> Mux/2
  FL Longitudinal force/1 -> Mux/3
  FL Lateral force/1 -> Mux/4
  RR Longitudinal force/1 -> Mux/5
  RR Lateral force/1 -> Mux/6
  RL Longitudinal force/1 -> Mux/7
  RL Lateral force/1 -> Mux/8
  Steering angle/1 -> Mux/9

== system AWD_EV_MODEL_rev2/Global Coordination Conversion ==
  Long. speed [m/s] : Inport
  Lateral speed [m/s] : Inport  Port=2
  Yaw angle [rad] : Inport  Port=3
  Fcn : Fcn  Expr=cos(u(3))*u(1)-sin(u(3))*u(2)
  Fcn1 : Fcn  Expr=sin(u(3))*u(1)+cos(u(3))*u(2)
  Integrator : Integrator
  Integrator1 : Integrator
  Mux : Mux  Inputs=3
  Long. distance [m] : Outport
  Lat. distance [m] : Outport  Port=2
  wires:
  Long. speed [m/s]/1 -> Mux/1
  Lateral speed [m/s]/1 -> Mux/2
  Yaw angle [rad]/1 -> Mux/3
  Mux/1 -> Fcn/1, Fcn1/1
  Fcn/1 -> Integrator/1
  Fcn1/1 -> Integrator1/1
  Integrator/1 -> Long. distance [m]/1
  Integrator1/1 -> Lat. distance [m]/1

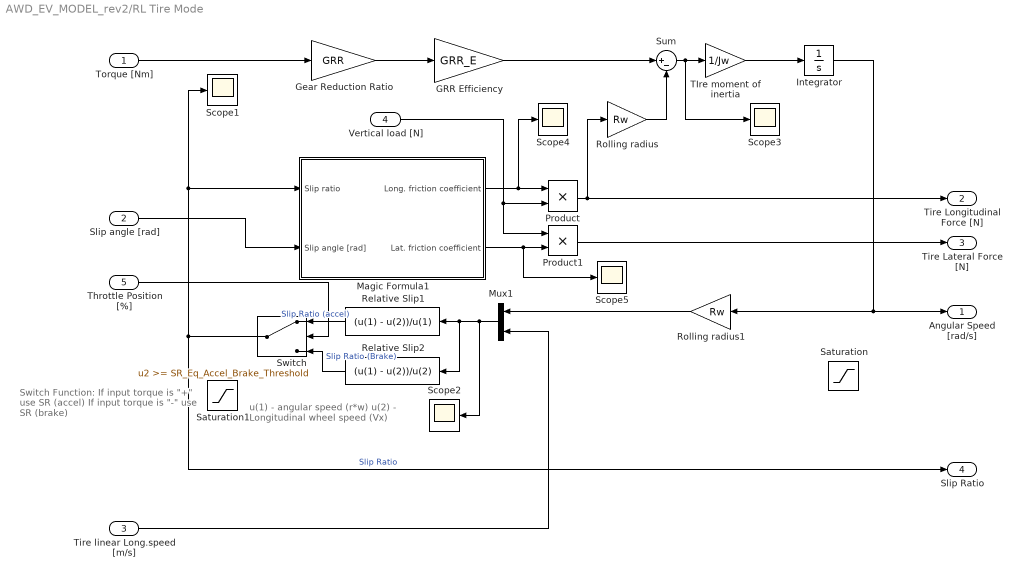
== system AWD_EV_MODEL_rev2/RL Tire Mode ==
  note: u(1) - angular speed (r*w)
      | u(2) - Longitudinal wheel speed (Vx)
  note: Switch Function:
      | If input torque is "+" use SR (accel)
      | If input torque is "-" use SR (brake)
  Torque [Nm] : Inport
  Slip angle [rad] : Inport  Port=2
  Tire linear Long.speed [m/s] : Inport  Port=3
  Vertical load [N] : Inport  Port=4
  Throttle Position [%] : Inport  Port=5
  GRR Efficiency : Gain  Gain=GRR_E  SaturateOnIntegerOverflow=on  OutDataTypeStr=Inherit: Same as input  ParamDataTypeStr=Inherit: Same as input
  Gear Reduction Ratio : Gain  Gain=GRR  SaturateOnIntegerOverflow=on  OutDataTypeStr=Inherit: Same as input  ParamDataTypeStr=Inherit: Same as input
  Integrator : Integrator  InitialCondition=wRL0
  Magic Formula1 : Subsystem  mask(Magic Formula (Combined Slip)){}
      mask Display:
      | image(imread('Magic formula.jpg'),'center')
      | port_label('input', 1, 'slip ratio')
      | port_label('input', 2, 'slip angle')
      | port_label('output', 1, 'Mux')
      | port_label('output', 2, 'Muy')
  Mux1 : Mux  Inputs=2
  Product : Product  RndMeth=Zero
  Product1 : Product  RndMeth=Zero
  Relative Slip1 : Fcn  Expr=(u(1) - u(2))/u(1)
  Relative Slip2 : Fcn  Expr=(u(1) - u(2))/u(2)
  Rolling radius : Gain  Gain=Rw  SaturateOnIntegerOverflow=on  OutDataTypeStr=Inherit: Same as input  ParamDataTypeStr=Inherit: Same as input
  Rolling radius1 : Gain  Gain=Rw  SaturateOnIntegerOverflow=on  OutDataTypeStr=Inherit: Same as input  ParamDataTypeStr=Inherit: Same as input
  Saturation : Saturate  UpperLimit=1000  LowerLimit=0.00001
  Saturation1 : Saturate  UpperLimit=1  LowerLimit=-1
  Scope{1..5} (5 alike) : Scope
  Sum : Sum  Inputs=|+-
  Switch : Switch  Threshold=SR_Eq_Accel_Brake_Threshold
  TIre moment of inertia : Gain  Gain=1/Jw  SaturateOnIntegerOverflow=on  OutDataTypeStr=Inherit: Same as input  ParamDataTypeStr=Inherit: Same as input
  Angular Speed [rad/s] : Outport
  Tire Longitudinal Force [N] : Outport  Port=2
  Tire Lateral Force [N] : Outport  Port=3
  Slip Ratio : Outport  Port=4
  wires:
  Slip angle [rad]/1 -> Magic Formula1/2(Slip angle [rad])
  Tire linear Long.speed [m/s]/1 -> Mux1/2
  Torque [Nm]/1 -> Gear Reduction Ratio/1
  Sum/1 -> TIre moment of inertia/1, Scope3/1
  TIre moment of inertia/1 -> Integrator/1
  Rolling radius/1 -> Sum/2
  Mux1/1 -> Scope2/1, Relative Slip1/1, Relative Slip2/1
  Rolling radius1/1 -> Mux1/1
  Magic Formula1/1(Long. friction coefficient) -> Product/1, Scope4/1
  Magic Formula1/2(Lat. friction coefficient) -> Product1/2, Scope5/1
  Product/1 -> Rolling radius/1, Tire Longitudinal Force [N]/1
  Vertical load [N]/1 -> Product/2, Product1/1
  Product1/1 -> Tire Lateral Force [N]/1
  Gear Reduction Ratio/1 -> GRR Efficiency/1
  GRR Efficiency/1 -> Sum/1
  Relative Slip1/1 -> Switch/1  "Slip Ratio (accel)"
  Relative Slip2/1 -> Switch/3  "Slip Ratio (Brake)"
  Switch/1 -> Magic Formula1/1(Slip ratio), Scope1/1, Slip Ratio/1  "Slip Ratio"
  Throttle Position [%]/1 -> Switch/2
  Integrator/1 -> Rolling radius1/1, Angular Speed [rad/s]/1

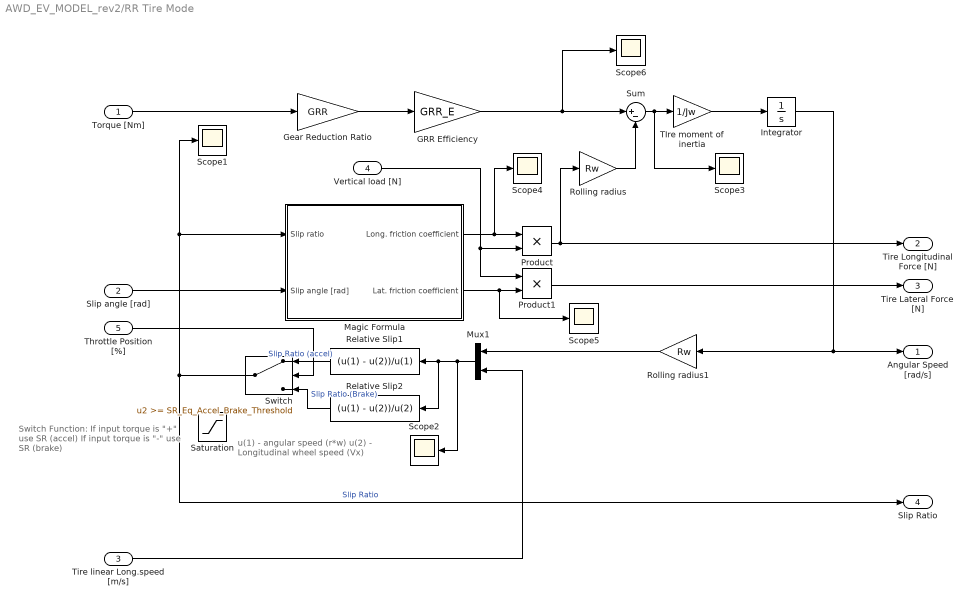
== system AWD_EV_MODEL_rev2/RR Tire Mode ==
  note: u(1) - angular speed (r*w)
      | u(2) - Longitudinal wheel speed (Vx)
  note: Switch Function:
      | If input torque is "+" use SR (accel)
      | If input torque is "-" use SR (brake)
  Torque [Nm] : Inport
  Slip angle [rad] : Inport  Port=2
  Tire linear Long.speed [m/s] : Inport  Port=3
  Vertical load [N] : Inport  Port=4
  Throttle Position [%] : Inport  Port=5
  GRR Efficiency : Gain  Gain=GRR_E  SaturateOnIntegerOverflow=on  OutDataTypeStr=Inherit: Same as input  ParamDataTypeStr=Inherit: Same as input
  Gear Reduction Ratio : Gain  Gain=GRR  SaturateOnIntegerOverflow=on  OutDataTypeStr=Inherit: Same as input  ParamDataTypeStr=Inherit: Same as input
  Integrator : Integrator  InitialCondition=wRL0
  Magic Formula : Subsystem  mask(Magic Formula (Combined Slip)){}
      mask Display:
      | image(imread('Magic formula.jpg'),'center')
      | port_label('input', 1, 'slip ratio')
      | port_label('input', 2, 'slip angle')
      | port_label('output', 1, 'Mux')
      | port_label('output', 2, 'Muy')
  Mux1 : Mux  Inputs=2
  Product : Product  RndMeth=Zero
  Product1 : Product  RndMeth=Zero
  Relative Slip1 : Fcn  Expr=(u(1) - u(2))/u(1)
  Relative Slip2 : Fcn  Expr=(u(1) - u(2))/u(2)
  Rolling radius : Gain  Gain=Rw  SaturateOnIntegerOverflow=on  OutDataTypeStr=Inherit: Same as input  ParamDataTypeStr=Inherit: Same as input
  Rolling radius1 : Gain  Gain=Rw  SaturateOnIntegerOverflow=on  OutDataTypeStr=Inherit: Same as input  ParamDataTypeStr=Inherit: Same as input
  Saturation : Saturate  UpperLimit=1  LowerLimit=-1
  Scope{1..6} (6 alike) : Scope
  Sum : Sum  Inputs=|+-
  Switch : Switch  Threshold=SR_Eq_Accel_Brake_Threshold
  TIre moment of inertia : Gain  Gain=1/Jw  SaturateOnIntegerOverflow=on  OutDataTypeStr=Inherit: Same as input  ParamDataTypeStr=Inherit: Same as input
  Angular Speed [rad/s] : Outport
  Tire Longitudinal Force [N] : Outport  Port=2
  Tire Lateral Force [N] : Outport  Port=3
  Slip Ratio : Outport  Port=4
  wires:
  Slip angle [rad]/1 -> Magic Formula/2(Slip angle [rad])
  Tire linear Long.speed [m/s]/1 -> Mux1/2
  Torque [Nm]/1 -> Gear Reduction Ratio/1
  Sum/1 -> TIre moment of inertia/1, Scope3/1
  TIre moment of inertia/1 -> Integrator/1
  Rolling radius/1 -> Sum/2
  Mux1/1 -> Scope2/1, Relative Slip1/1, Relative Slip2/1
  Rolling radius1/1 -> Mux1/1
  Magic Formula/1(Long. friction coefficient) -> Product/1, Scope4/1
  Magic Formula/2(Lat. friction coefficient) -> Product1/2, Scope5/1
  Product/1 -> Rolling radius/1, Tire Longitudinal Force [N]/1
  Vertical load [N]/1 -> Product/2, Product1/1
  Product1/1 -> Tire Lateral Force [N]/1
  Gear Reduction Ratio/1 -> GRR Efficiency/1
  GRR Efficiency/1 -> Scope6/1, Sum/1
  Relative Slip1/1 -> Switch/1  "Slip Ratio (accel)"
  Relative Slip2/1 -> Switch/3  "Slip Ratio (Brake)"
  Switch/1 -> Magic Formula/1(Slip ratio), Scope1/1, Slip Ratio/1  "Slip Ratio"
  Throttle Position [%]/1 -> Switch/2
  Integrator/1 -> Rolling radius1/1, Angular Speed [rad/s]/1

== system AWD_EV_MODEL_rev2/Signal Builder ==
  Demux : Demux  Tag=STV Demux  Outputs=1
  FromWs : FromWorkspace  Tag=STV FromWs  VariableName=tuvar  SampleTime=0  SigBuilderData=DataTag0  VnvData=DataTag1
      SigBuilderData=|
      | common.afterFinalStr = 'Extrapolate'
      | common.sampleTime = 0
      | dataSet.timeRange = [0 3]
      | dataSet.name = 'Group 1'
      | sbobj.Groups.Name = 'Group 1'
      | sbobj.Groups.Signals.Name = 'Signal 1'
      | sbobj.Groups.Signals.XData = [0 0.0492610837438 0.0985221674877 0.147783251232 0.197044334975 0.246305418719 0.295566502463 0.344827586207 0.394088669951 0.443349753695 0.492610837438 0.541871921182 0.591133004926 0.64039408867 0.689655172414 0.738916256158 0.788177339901 0.837438423645 0.886699507389 0.935960591133 0.985221674877 1.03448275862 1.08374384236 1.13300492611 1.18226600985 1.2315270936 1.28078817734 1.33004926108 1.37931034483 1.42857142857 1.47783251232 1.52709359606 1.5763546798 1.62561576355 1.67487684729 1.72413793103 1.77339901478 1.82266009852 1.87192118227 1.92118226601 1.97044334975 2 3]
      | sbobj.Groups.Signals.YData = [1 1.21497044021 1.41988910156 1.60517421519 1.76216205513 1.88351204445 1.96354999252 1.99853341385 1.98682652254 1.92897671982 1.82768899816 1.68769945885 1.5 1.31930153014 1.10811901842 0.891880981576 0.680698469864 0.484446142823 0.312300541147 0.172311001843 0.0710232801832 0.0131734774585 0.00146658614888 0 0 0 0 0 0 0 0 0 0 0.0132 0.071 0.1723 0.3123 0.5 0.72 1 1 1 1]
      | sbobj.Groups.TimeRange = [0 3]
  Signal 1 : Outport  Tag=STV Outport
  wires:
  Demux/1 -> Signal 1/1
  FromWs/1 -> Demux/1

== system AWD_EV_MODEL_rev2/Signal Builder1 ==
  Demux : Demux  Tag=STV Demux  Outputs=1
  FromWs : FromWorkspace  Tag=STV FromWs  VariableName=tuvar  SampleTime=0  SigBuilderData=DataTag2  VnvData=DataTag3
      SigBuilderData=|
      | common.afterFinalStr = 'Extrapolate'
      | common.sampleTime = 0
      | dataSet.timeRange = [0 15]
      | dataSet.name = 'Group 1'
      | sbobj.Groups.Name = 'Group 1'
      | sbobj.Groups.Signals.Name = 'Signal 1'
      | sbobj.Groups.Signals.XData = [0 0.125 0.25 0.375 0.5 0.625 0.75 0.875 1 1.125 1.25 1.375 1.5 1.625 1.75 1.875 2 2.125 2.25 2.375 2.5 2.625 2.75 2.875 3 3.125 3.25 3.375 3.5 3.625 3.75 3.75 3.875 3.875 4 4.125 4.25 4.375 4.5 4.625 4.75 4.875 5 5.125 5.25 5.375 5.5 5.625 5.75 5.875 6 6.125 6.25 6.375 6.5 6.625 6.75 6.875 7 7.125 7.25 7.375 7.5 7.625 7.75 7.875 8 8.125 8.25 8.375 8.5 8.625 8.75 8.875 9 9.125 9.25 9.375 9.5 9.625 9.75 9.875 10 10.125 10.25 10.375 10.5 10.625 10.75 10.875 11 11.125 11.25 11.375 11.5 11.625 11.75 11.875 12 12.125 12.25 12.375 12.5 12.625 12.75 12.875 13 13.125 13.25 13.375 13.5 13.625 13.75 13.875 14 14.125 14.25 14.375 14.5 14.625 14.75 14.875 15]
      | sbobj.Groups.Signals.YData = [1 1.70710678119 2 1.70710678119 1 0.292893218813 0 0.292893218813 1 1.70710678119 2 1.70710678119 1 0.292893218813 0 0.292893218813 1 1.70710678119 2 1.70710678119 1 0.292893218813 0 0.292893218813 1 1.70710678119 2 1.70710678119 1 0.292893218813 -0.355 -0.335 -0.36 0.985 1 1.70710678119 2 1.70710678119 1 0.292893218813 0 0.292893218813 1 1.70710678119 2 1.70710678119 1 0.292893218813 0 0.292893218813 1 1.70710678119 2 1.70710678119 1 0.292893218813 0 0.292893218813 1 1.70710678119 2 1.70710678119 1 0.292893218813 0 0.292893218813 1 1.70710678119 2 1.70710678119 1 0.292893218813 0 0.292893218813 1 1.70710678119 2 1.70710678119 1 0.292893218813 0 0.292893218813 1 1.70710678119 2 1.70710678119 1 0.292893218813 0 0.292893218813 1 1.70710678119 2 1.70710678119 1 0.292893218813 0 0.292893218813 1 1.70710678119 2 1.70710678119 1 0.292893218813 0 0.292893218813 1 1.70710678119 2 1.70710678119 1 0.292893218813 0 0.292893218813 1 1.70710678119 2 1.70710678119 1 0.292893218813 0 0.292893218813 1]
      | sbobj.Groups.TimeRange = [0 15]
  Signal 1 : Outport  Tag=STV Outport
  wires:
  Demux/1 -> Signal 1/1
  FromWs/1 -> Demux/1

== system AWD_EV_MODEL_rev2/Signal Builder2 ==
  Demux : Demux  Tag=STV Demux  Outputs=1
  FromWs : FromWorkspace  Tag=STV FromWs  VariableName=tuvar  SampleTime=0  SigBuilderData=DataTag4  VnvData=DataTag5
      SigBuilderData=|
      | common.afterFinalStr = 'Extrapolate'
      | common.sampleTime = 0
      | dataSet.timeRange = [0 3]
      | dataSet.name = 'Group 1'
      | sbobj.Groups.Name = 'Group 1'
      | sbobj.Groups.Signals.Name = 'Signal 1'
      | sbobj.Groups.Signals.XData = [0 0.0492610837438 0.0985221674877 0.147783251232 0.197044334975 0.246305418719 0.295566502463 0.344827586207 0.394088669951 0.443349753695 0.492610837438 0.541871921182 0.591133004926 0.64039408867 0.689655172414 0.738916256158 0.788177339901 0.837438423645 0.886699507389 0.935960591133 0.985221674877 1.03448275862 1.08374384236 1.13300492611 1.18226600985 1.2315270936 1.28078817734 1.33004926108 1.37931034483 1.42857142857 1.47783251232 1.52709359606 1.5763546798 1.62561576355 1.67487684729 1.72413793103 1.77339901478 1.82266009852 1.87192118227 1.92118226601 1.97044334975 2 3]
      | sbobj.Groups.Signals.YData = [1 1.075 1.145 1.185 1.21 1.24 1.25 1.225 1.2 1.17 1.145 1.1 1.05 1.02 0.955 0.891880981576 0.680698469864 0.484446142823 0.312300541147 0.172311001843 0.0710232801832 0.0131734774585 0.00146658614888 0 0 0 0 0 0 0 0 0 0 0.0132 0.071 0.1723 0.3123 0.5 0.72 0.975 1 1 1]
      | sbobj.Groups.TimeRange = [0 3]
  Signal 1 : Outport  Tag=STV Outport
  wires:
  Demux/1 -> Signal 1/1
  FromWs/1 -> Demux/1

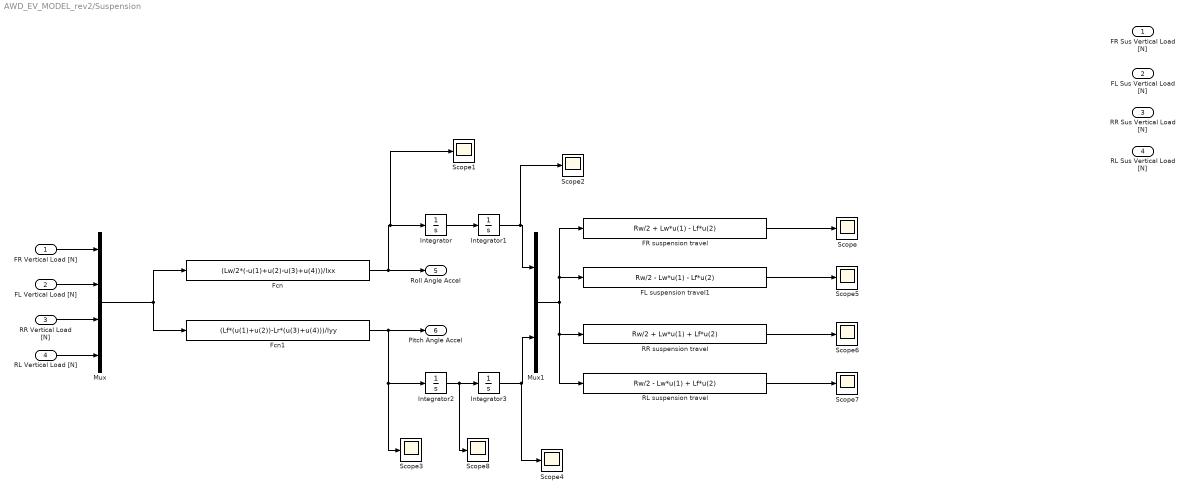
== system AWD_EV_MODEL_rev2/Suspension ==
  FR Vertical Load [N] : Inport
  FL Vertical Load [N] : Inport  Port=2
  RR Vertical Load [N] : Inport  Port=3
  RL Vertical Load [N] : Inport  Port=4
  FL suspension travel1 : Fcn  Expr=Rw/2 - Lw*u(1) - Lf*u(2)
  FR suspension travel : Fcn  Expr=Rw/2 + Lw*u(1) - Lf*u(2)
  Fcn : Fcn  Expr=(Lw/2*(-u(1)+u(2)-u(3)+u(4)))/Ixx
  Fcn1 : Fcn  Expr=(Lf*(u(1)+u(2))-Lr*(u(3)+u(4)))/Iyy
  Integrator{,1..3} (4 alike) : Integrator
  Mux : Mux
  Mux1 : Mux  Inputs=2
  RL suspension travel : Fcn  Expr=Rw/2 - Lw*u(1) + Lf*u(2)
  RR suspension travel : Fcn  Expr=Rw/2 + Lw*u(1) + Lf*u(2)
  Scope{,1..8} (9 alike) : Scope
  FR Sus Vertical Load [N] : Outport
  FL Sus Vertical Load [N] : Outport  Port=2
  RR Sus Vertical Load [N] : Outport  Port=3
  RL Sus Vertical Load [N] : Outport  Port=4
  Roll Angle Accel : Outport  Port=5
  Pitch Angle Accel : Outport  Port=6
  wires:
  RR Vertical Load [N]/1 -> Mux/3
  FL Vertical Load [N]/1 -> Mux/2
  FR Vertical Load [N]/1 -> Mux/1
  RL Vertical Load [N]/1 -> Mux/4
  ? -> FR Sus Vertical Load [N]/1
  ? -> FL Sus Vertical Load [N]/1
  ? -> RR Sus Vertical Load [N]/1
  ? -> RL Sus Vertical Load [N]/1
  Mux/1 -> Fcn1/1, Fcn/1
  Fcn/1 -> Roll Angle Accel/1, Scope1/1, Integrator/1
  Integrator/1 -> Integrator1/1
  Fcn1/1 -> Scope3/1, Integrator2/1, Pitch Angle Accel/1
  Integrator2/1 -> Scope8/1, Integrator3/1
  Integrator1/1 -> Scope2/1, Mux1/1
  Integrator3/1 -> Scope4/1, Mux1/2
  Mux1/1 -> RR suspension travel/1, RL suspension travel/1, FL suspension travel1/1, FR suspension travel/1
  FR suspension travel/1 -> Scope/1
  FL suspension travel1/1 -> Scope5/1
  RR suspension travel/1 -> Scope6/1
  RL suspension travel/1 -> Scope7/1

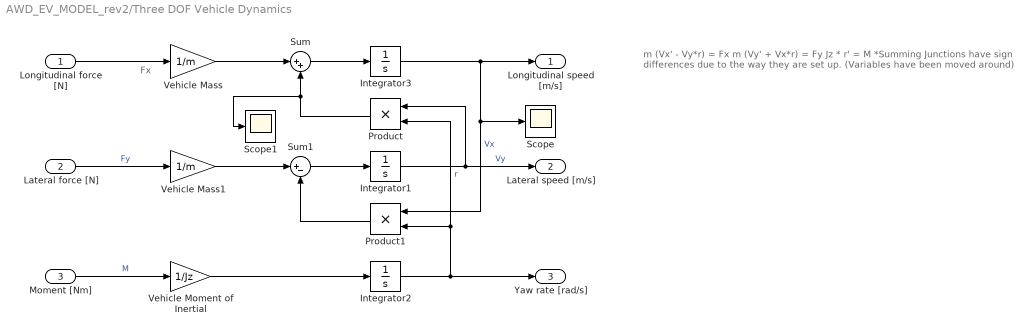
== system AWD_EV_MODEL_rev2/Three DOF Vehicle Dynamics ==
  note: m (Vx' - Vy*r) = Fx
      | m (Vy' + Vx*r) = Fy
      |
      | Jz * r' = M
      |
      | *Summing Junctions have sign differences due to
      | the way they are set up. (Variables have been moved around)
  note: Fx
  Longitudinal force [N] : Inport
  Lateral force [N] : Inport  Port=2
  Moment [Nm] : Inport  Port=3
  Integrator1 : Integrator  InitialCondition=Vy0  UpperSaturationLimit=1000  LowerSaturationLimit=0
  Integrator2 : Integrator  InitialCondition=r0
  Integrator3 : Integrator  InitialCondition=Vx0  UpperSaturationLimit=1000  LowerSaturationLimit=0
  Product : Product  RndMeth=Zero
  Product1 : Product  RndMeth=Zero
  Scope : Scope
  Scope1 : Scope
  Sum : Sum  Inputs=|++
  Sum1 : Sum  Inputs=|+-
  Vehicle Mass : Gain  Gain=1/m
  Vehicle Mass1 : Gain  Gain=1/m
  Vehicle Moment of Inertial : Gain  Gain=1/Jz
  Longitudinal speed [m/s] : Outport
  Lateral speed [m/s] : Outport  Port=2
  Yaw rate [rad/s] : Outport  Port=3
  wires:
  Integrator2/1 -> Yaw rate [rad/s]/1, Product/2, Product1/2  "r"
  Moment [Nm]/1 -> Vehicle Moment of Inertial/1  "M"
  Integrator1/1 -> Product/1, Lateral speed [m/s]/1  "Vy"
  Integrator3/1 -> Longitudinal speed [m/s]/1, Product1/1, Scope/1  "Vx"
  Vehicle Moment of Inertial/1 -> Integrator2/1
  Vehicle Mass1/1 -> Sum1/1
  Lateral force [N]/1 -> Vehicle Mass1/1  "Fy"
  Vehicle Mass/1 -> Sum/1
  Sum1/1 -> Integrator1/1
  Product1/1 -> Sum1/2
  Sum/1 -> Integrator3/1
  Product/1 -> Sum/2, Scope1/1
  Longitudinal force [N]/1 -> Vehicle Mass/1

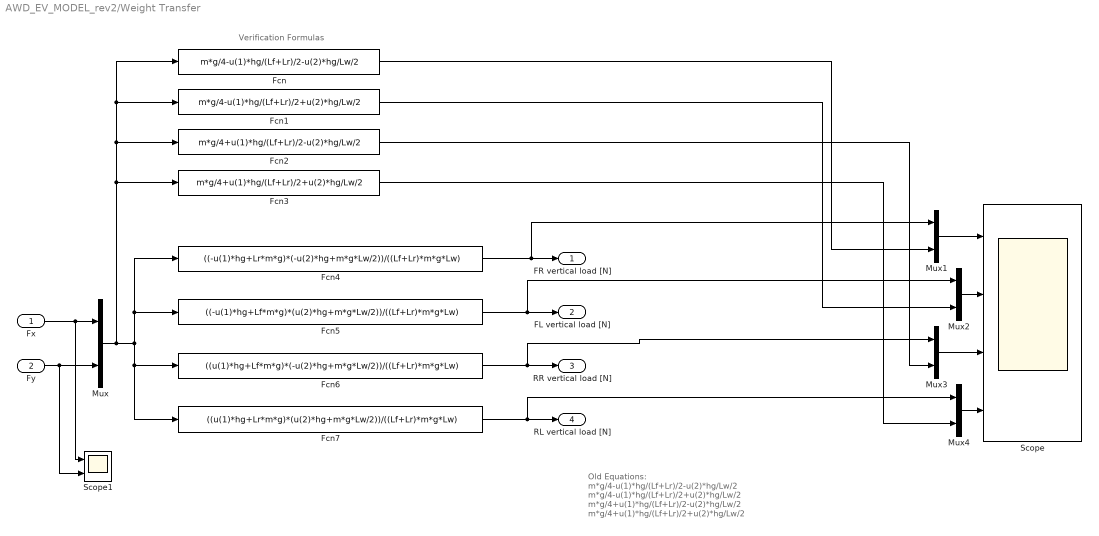
== system AWD_EV_MODEL_rev2/Weight Transfer ==
  note: Old Equations:
      | m*g/4-u(1)*hg/(Lf+Lr)/2-u(2)*hg/Lw/2
      | m*g/4-u(1)*hg/(Lf+Lr)/2+u(2)*hg/Lw/2
      | m*g/4+u(1)*hg/(Lf+Lr)/2-u(2)*hg/Lw/2
      | m*g/4+u(1)*hg/(Lf+Lr)/2+u(2)*hg/Lw/2
  note: Verification Formulas
  Fx : Inport
  Fy : Inport  Port=2
  Fcn : Fcn  Expr=m*g/4-u(1)*hg/(Lf+Lr)/2-u(2)*hg/Lw/2
  Fcn1 : Fcn  Expr=m*g/4-u(1)*hg/(Lf+Lr)/2+u(2)*hg/Lw/2
  Fcn2 : Fcn  Expr=m*g/4+u(1)*hg/(Lf+Lr)/2-u(2)*hg/Lw/2
  Fcn3 : Fcn  Expr=m*g/4+u(1)*hg/(Lf+Lr)/2+u(2)*hg/Lw/2
  Fcn4 : Fcn  Expr=((-u(1)*hg+Lr*m*g)*(-u(2)*hg+m*g*Lw/2))/((Lf+Lr)*m*g*Lw)
  Fcn5 : Fcn  Expr=((-u(1)*hg+Lf*m*g)*(u(2)*hg+m*g*Lw/2))/((Lf+Lr)*m*g*Lw)
  Fcn6 : Fcn  Expr=((u(1)*hg+Lf*m*g)*(-u(2)*hg+m*g*Lw/2))/((Lf+Lr)*m*g*Lw)
  Fcn7 : Fcn  Expr=((u(1)*hg+Lr*m*g)*(u(2)*hg+m*g*Lw/2))/((Lf+Lr)*m*g*Lw)
  Mux{,1..4} (5 alike) : Mux  Inputs=2
  Scope : Scope  NumInputPorts=4
  Scope1 : Scope  NumInputPorts=2
  FR vertical load [N] : Outport
  FL vertical load [N] : Outport  Port=2
  RR vertical load [N] : Outport  Port=3
  RL vertical load [N] : Outport  Port=4
  wires:
  Fy/1 -> Scope1/2, Mux/2
  Fx/1 -> Scope1/1, Mux/1
  Fcn4/1 -> Mux1/1, FR vertical load [N]/1
  Fcn5/1 -> Mux2/1, FL vertical load [N]/1
  Fcn6/1 -> Mux3/1, RR vertical load [N]/1
  Fcn7/1 -> Mux4/1, RL vertical load [N]/1
  Fcn/1 -> Mux1/2
  Fcn1/1 -> Mux2/2
  Fcn2/1 -> Mux3/2
  Fcn3/1 -> Mux4/2
  Mux/1 -> Fcn4/1, Fcn5/1, Fcn6/1, Fcn7/1, Fcn3/1, Fcn2/1, Fcn1/1, Fcn/1
  Mux1/1 -> Scope/1
  Mux2/1 -> Scope/2
  Mux3/1 -> Scope/3
  Mux4/1 -> Scope/4

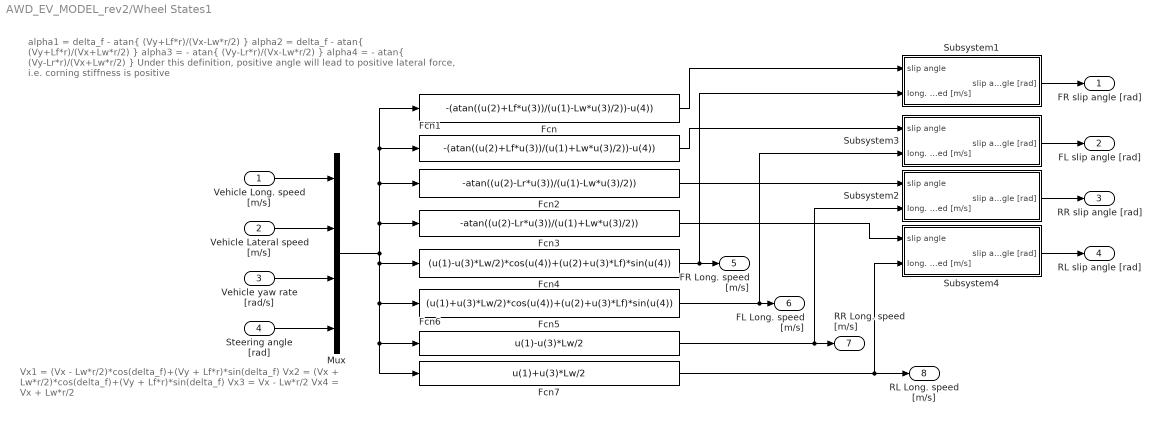
== system AWD_EV_MODEL_rev2/Wheel States1 ==
  note: alpha1 = delta_f - atan{ (Vy+Lf*r)/(Vx-Lw*r/2) }
      | alpha2 = delta_f - atan{ (Vy+Lf*r)/(Vx+Lw*r/2) }
      | alpha3 = - atan{ (Vy-Lr*r)/(Vx-Lw*r/2) }
      | alpha4 = - atan{ (Vy-Lr*r)/(Vx+Lw*r/2) }
      | Under this definition, positive angle will lead to  positive lateral force,
      | i.e. corning stiffness is positive
  note: Vx1 = (Vx - Lw*r/2)*cos(delta_f)+(Vy + Lf*r)*sin(delta_f)
      | Vx2 = (Vx + Lw*r/2)*cos(delta_f)+(Vy + Lf*r)*sin(delta_f)
      | Vx3 = Vx - Lw*r/2
      | Vx4 = Vx + Lw*r/2
  Vehicle Long. speed [m/s] : Inport
  Vehicle Lateral speed [m/s] : Inport  Port=2
  Vehicle yaw rate [rad/s] : Inport  Port=3
  Steering angle [rad] : Inport  Port=4
  Fcn : Fcn  Expr=-(atan((u(2)+Lf*u(3))/(u(1)-Lw*u(3)/2))-u(4))
  Fcn1 : Fcn  Expr=-(atan((u(2)+Lf*u(3))/(u(1)+Lw*u(3)/2))-u(4))
  Fcn2 : Fcn  Expr=-atan((u(2)-Lr*u(3))/(u(1)-Lw*u(3)/2))
  Fcn3 : Fcn  Expr=-atan((u(2)-Lr*u(3))/(u(1)+Lw*u(3)/2))
  Fcn4 : Fcn  Expr=(u(1)-u(3)*Lw/2)*cos(u(4))+(u(2)+u(3)*Lf)*sin(u(4))
  Fcn5 : Fcn  Expr=(u(1)+u(3)*Lw/2)*cos(u(4))+(u(2)+u(3)*Lf)*sin(u(4))
  Fcn6 : Fcn  Expr=u(1)-u(3)*Lw/2
  Fcn7 : Fcn  Expr=u(1)+u(3)*Lw/2
  Mux : Mux
  Subsystem1 : Subsystem
  Subsystem2 : Subsystem
  Subsystem3 : Subsystem
  Subsystem4 : Subsystem
  "FR slip angle [rad] " : Outport
  "FL slip angle [rad] " : Outport  Port=2
  "RR slip angle [rad] " : Outport  Port=3
  "RL slip angle [rad] " : Outport  Port=4
  FR Long. speed [m/s] : Outport  Port=5
  FL Long. speed [m/s] : Outport  Port=6
  RR Long. speed [m/s] : Outport  Port=7
  RL Long. speed [m/s] : Outport  Port=8
  wires:
  Vehicle yaw rate [rad/s]/1 -> Mux/3
  Vehicle Lateral speed [m/s]/1 -> Mux/2
  Vehicle Long. speed [m/s]/1 -> Mux/1
  Steering angle [rad]/1 -> Mux/4
  Fcn4/1 -> FR Long. speed [m/s]/1, Subsystem1/2(long. speed [m/s])
  Fcn5/1 -> FL Long. speed [m/s]/1, Subsystem3/2(long. speed [m/s])
  Fcn6/1 -> RR Long. speed [m/s]/1, Subsystem2/2(long. speed [m/s])
  Fcn7/1 -> RL Long. speed [m/s]/1, Subsystem4/2(long. speed [m/s])
  Mux/1 -> Fcn5/1, Fcn7/1, Fcn6/1, Fcn4/1, Fcn3/1, Fcn2/1, Fcn1/1, Fcn/1
  Subsystem1/1(slip angle [rad]) -> "FR slip angle [rad] "/1
  Fcn/1 -> Subsystem1/1(slip angle)
  Subsystem3/1(slip angle [rad]) -> "FL slip angle [rad] "/1
  Fcn1/1 -> Subsystem3/1(slip angle)
  Fcn2/1 -> Subsystem2/1(slip angle)
  Fcn3/1 -> Subsystem4/1(slip angle)
  Subsystem2/1(slip angle [rad]) -> "RR slip angle [rad] "/1
  Subsystem4/1(slip angle [rad]) -> "RL slip angle [rad] "/1

== system AWD_EV_MODEL_rev2/FL Tire Mode/Magic Formula ==
  Slip ratio : Inport
  Slip angle [rad] : Inport  Port=2
  Digital Clock : DigitalClock  SampleTime=0.001
  Magic Formula Condition 1 : Subsystem
  Magic Formula Condition 2 : Subsystem
  Repeating Sequence Interpolated1 : simulink/Sources/Repeating Sequence Interpolated  OutValues=[0 0 5 5 0 0 5 5 0 0 5 5 0 0].'  TimeValues=[0 1 1.001 1.5 1.501 3 3.001 3.5 3.501 5 5.001 5.5 5.501 10].'  LookUpMeth=Interpolation-Use End Values  tsamp=0.001  OutMin=[]  OutMax=[]  OutDataTypeStr=double  OutputDataTypeScalingMode=double  OutDataType=fixdt(0,8)  OutScaling=2^-10
  Repeating Sequence Interpolated2 : simulink/Sources/Repeating Sequence Interpolated  OutValues=[0 0 5 5 0 0 5 5 0 0 0 0 0 0].'  TimeValues=[0 1 1.001 1.5 1.501 3 3.001 3.5 3.501 5 5.001 5.5 5.501 10].'  LookUpMeth=Interpolation-Use End Values  tsamp=0.001  OutMin=[]  OutMax=[]  OutDataTypeStr=double  OutputDataTypeScalingMode=double  OutDataType=fixdt(0,8)  OutScaling=2^-10
  Scope : Scope
  Scope1 : Scope
  Scope2 : Scope
  Switch : Switch  Criteria=u2 > Threshold  Threshold=Split_u_Time_On
  Switch1 : Switch  Criteria=u2 > Threshold  Threshold=Split_u_Time_On
  Long. friction coefficient : Outport
  Lat. friction coefficient : Outport  Port=2
  wires:
  Slip ratio/1 -> Magic Formula Condition 2/1(Slip ratio), Magic Formula Condition 1/1(Slip ratio)
  Slip angle [rad]/1 -> Magic Formula Condition 2/2(Slip angle [rad]), Magic Formula Condition 1/2(Slip angle [rad])
  Switch/1 -> Long. friction coefficient/1
  Switch1/1 -> Lat. friction coefficient/1
  Magic Formula Condition 2/1(Long. friction coefficient) -> Switch/1, Scope1/1
  Magic Formula Condition 1/1(Long. friction coefficient) -> Scope/1, Switch/3
  Magic Formula Condition 1/2(Lat. friction coefficient) -> Switch1/3
  Magic Formula Condition 2/2(Lat. friction coefficient) -> Switch1/1
  Digital Clock/1 -> Scope2/1, Switch1/2, Switch/2

== system AWD_EV_MODEL_rev2/FR Tire Mode/Magic Formula1 ==
  Slip ratio : Inport
  Slip angle [rad] : Inport  Port=2
  Digital Clock1 : DigitalClock  SampleTime=0.001
  Magic Formula Condition 1 : Subsystem
  Magic Formula Condition 2 : Subsystem
  Repeating Sequence Interpolated1 : simulink/Sources/Repeating Sequence Interpolated  OutValues=[0 0 5 5 0 0 5 5 0 0 0 0 0 0].'  TimeValues=[0 1 1.001 1.5 1.501 3 3.001 3.5 3.501 5 5.001 5.5 5.501 10].'  LookUpMeth=Interpolation-Use End Values  tsamp=0.001  OutMin=[]  OutMax=[]  OutDataTypeStr=double  OutputDataTypeScalingMode=double  OutDataType=fixdt(0,8)  OutScaling=2^-10
  Repeating Sequence Interpolated2 : simulink/Sources/Repeating Sequence Interpolated  OutValues=[0 0 5 5 0 0 5 5 0 0 5 5 0 0].'  TimeValues=[0 1 1.001 1.5 1.501 3 3.001 3.5 3.501 5 5.001 5.5 5.501 10].'  LookUpMeth=Interpolation-Use End Values  tsamp=0.001  OutMin=[]  OutMax=[]  OutDataTypeStr=double  OutputDataTypeScalingMode=double  OutDataType=fixdt(0,8)  OutScaling=2^-10
  Scope2 : Scope
  Switch : Switch  Criteria=u2 > Threshold  Threshold=Split_u_Time_On
  Switch1 : Switch  Criteria=u2 > Threshold  Threshold=Split_u_Time_On
  Long. friction coefficient : Outport
  Lat. friction coefficient : Outport  Port=2
  wires:
  Slip ratio/1 -> Magic Formula Condition 2/1(Slip ratio), Magic Formula Condition 1/1(Slip ratio)
  Slip angle [rad]/1 -> Magic Formula Condition 2/2(Slip angle [rad]), Magic Formula Condition 1/2(Slip angle [rad])
  Switch/1 -> Long. friction coefficient/1
  Switch1/1 -> Lat. friction coefficient/1
  Magic Formula Condition 2/1(Long. friction coefficient) -> Switch/1
  Magic Formula Condition 1/1(Long. friction coefficient) -> Switch/3
  Magic Formula Condition 1/2(Lat. friction coefficient) -> Switch1/3
  Magic Formula Condition 2/2(Lat. friction coefficient) -> Switch1/1
  Digital Clock1/1 -> Switch1/2, Switch/2, Scope2/1

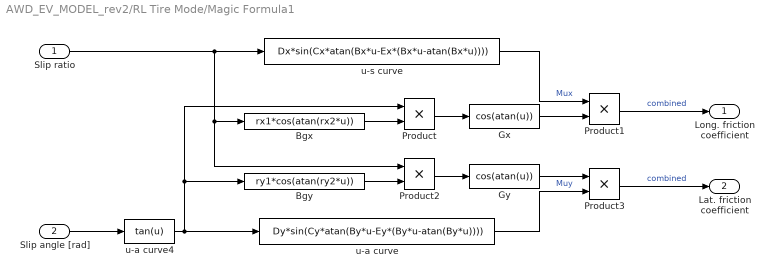
== system AWD_EV_MODEL_rev2/RL Tire Mode/Magic Formula1 ==
  Slip ratio : Inport
  Slip angle [rad] : Inport  Port=2
  Bgx : Fcn  Expr=rx1*cos(atan(rx2*u))
  Bgy : Fcn  Expr=ry1*cos(atan(ry2*u))
  Gx : Fcn  Expr=cos(atan(u))
  Gy : Fcn  Expr=cos(atan(u))
  Product{,1..3} (4 alike) : Product  RndMeth=Zero
  u-a curve : Fcn  Expr=Dy*sin(Cy*atan(By*u-Ey*(By*u-atan(By*u))))
  u-a curve4 : Fcn  Expr=tan(u)
  u-s curve : Fcn  Expr=Dx*sin(Cx*atan(Bx*u-Ex*(Bx*u-atan(Bx*u))))
  Long. friction coefficient : Outport
  Lat. friction coefficient : Outport  Port=2
  wires:
  Bgx/1 -> Product/2
  Bgy/1 -> Product2/2
  Slip angle [rad]/1 -> u-a curve4/1
  Product3/1 -> Lat. friction coefficient/1  "combined"
  Gy/1 -> Product3/1
  Product2/1 -> Gy/1
  Product1/1 -> Long. friction coefficient/1  "combined"
  Gx/1 -> Product1/2
  Product/1 -> Gx/1
  u-a curve4/1 -> Product/1, Bgy/1, u-a curve/1
  Slip ratio/1 -> Bgx/1, Product2/1, u-s curve/1
  u-a curve/1 -> Product3/2  "Muy"
  u-s curve/1 -> Product1/1  "Mux"

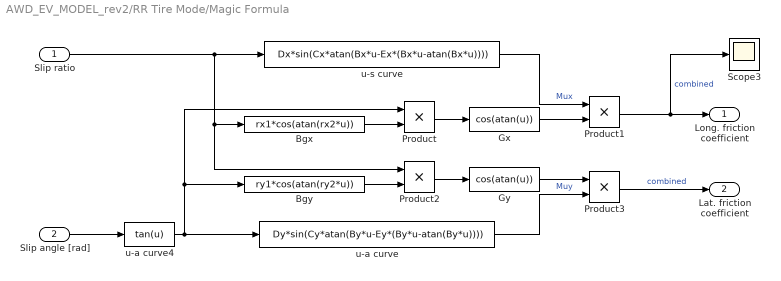
== system AWD_EV_MODEL_rev2/RR Tire Mode/Magic Formula ==
  Slip ratio : Inport
  Slip angle [rad] : Inport  Port=2
  Bgx : Fcn  Expr=rx1*cos(atan(rx2*u))
  Bgy : Fcn  Expr=ry1*cos(atan(ry2*u))
  Gx : Fcn  Expr=cos(atan(u))
  Gy : Fcn  Expr=cos(atan(u))
  Product{,1..3} (4 alike) : Product  RndMeth=Zero
  Scope3 : Scope
  u-a curve : Fcn  Expr=Dy*sin(Cy*atan(By*u-Ey*(By*u-atan(By*u))))
  u-a curve4 : Fcn  Expr=tan(u)
  u-s curve : Fcn  Expr=Dx*sin(Cx*atan(Bx*u-Ex*(Bx*u-atan(Bx*u))))
  Long. friction coefficient : Outport
  Lat. friction coefficient : Outport  Port=2
  wires:
  Bgx/1 -> Product/2
  Bgy/1 -> Product2/2
  Slip angle [rad]/1 -> u-a curve4/1
  Product3/1 -> Lat. friction coefficient/1  "combined"
  Gy/1 -> Product3/1
  Product2/1 -> Gy/1
  Product1/1 -> Scope3/1, Long. friction coefficient/1  "combined"
  Gx/1 -> Product1/2
  Product/1 -> Gx/1
  u-a curve4/1 -> Product/1, Bgy/1, u-a curve/1
  Slip ratio/1 -> Bgx/1, Product2/1, u-s curve/1
  u-a curve/1 -> Product3/2  "Muy"
  u-s curve/1 -> Product1/1  "Mux"

== system AWD_EV_MODEL_rev2/Wheel States1/Subsystem1 ==
  slip angle : Inport
  long. speed [m/s] : Inport  Port=2
  If : If
  Merge1 : Merge
  negative slip angle : Subsystem  TreatAsAtomicUnit=on
  positive slip angle : Subsystem  TreatAsAtomicUnit=on
  slip angle [rad] : Outport
  wires:
  If/2 -> negative slip angle/Action
  negative slip angle/1(-in) -> Merge1/2
  positive slip angle/1(+in) -> Merge1/1
  If/1 -> positive slip angle/Action
  long. speed [m/s]/1 -> If/1
  slip angle/1 -> negative slip angle/1(in), positive slip angle/1(in)
  Merge1/1 -> slip angle [rad]/1

== system AWD_EV_MODEL_rev2/Wheel States1/Subsystem2 ==
  slip angle : Inport
  long. speed [m/s] : Inport  Port=2
  If : If
  Merge1 : Merge
  negative slip angle : Subsystem  TreatAsAtomicUnit=on
  positive slip angle : Subsystem  TreatAsAtomicUnit=on
  slip angle [rad] : Outport
  wires:
  Merge1/1 -> slip angle [rad]/1
  slip angle/1 -> positive slip angle/1(in), negative slip angle/1(in)
  long. speed [m/s]/1 -> If/1
  If/1 -> positive slip angle/Action
  positive slip angle/1(+in) -> Merge1/1
  negative slip angle/1(-in) -> Merge1/2
  If/2 -> negative slip angle/Action

== system AWD_EV_MODEL_rev2/Wheel States1/Subsystem3 ==
  slip angle : Inport
  long. speed [m/s] : Inport  Port=2
  If : If
  Merge1 : Merge
  negative slip angle : Subsystem  TreatAsAtomicUnit=on
  positive slip angle : Subsystem  TreatAsAtomicUnit=on
  slip angle [rad] : Outport
  wires:
  Merge1/1 -> slip angle [rad]/1
  slip angle/1 -> positive slip angle/1(in), negative slip angle/1(in)
  long. speed [m/s]/1 -> If/1
  If/1 -> positive slip angle/Action
  positive slip angle/1(+in) -> Merge1/1
  negative slip angle/1(-in) -> Merge1/2
  If/2 -> negative slip angle/Action

== system AWD_EV_MODEL_rev2/Wheel States1/Subsystem4 ==
  slip angle : Inport
  long. speed [m/s] : Inport  Port=2
  If : If
  Merge1 : Merge
  negative slip angle : Subsystem  TreatAsAtomicUnit=on
  positive slip angle : Subsystem  TreatAsAtomicUnit=on
  slip angle [rad] : Outport
  wires:
  If/2 -> negative slip angle/Action
  negative slip angle/1(-in) -> Merge1/2
  positive slip angle/1(+in) -> Merge1/1
  If/1 -> positive slip angle/Action
  long. speed [m/s]/1 -> If/1
  slip angle/1 -> negative slip angle/1(in), positive slip angle/1(in)
  Merge1/1 -> slip angle [rad]/1
